simulink model "SNS_W2L_CPG"  (R2025b)
settings: Solver=ode1  StartTime=0.0  StopTime=10.0  FixedStep=0.002  RelTol=1e-3
libraries: SNS_Library x64
Description:
  | SNS_W2L_CPG: representative core of the W2L contact-driven bilateral CPG (build_w2l_net.py), SNS_Library blocks + custom NapHC (persistent Na, fixed tau_h). Validated against the numpy reference campaigns/20260930/w2l_numpy_ref.json.
settings Model: Creator=Ben  LastModifiedBy=Ben

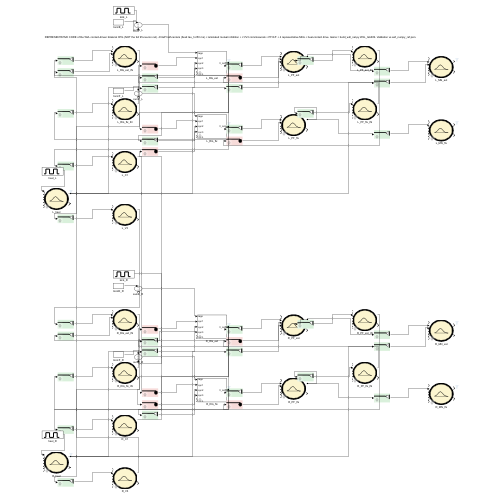
[thumbnail: Simulink's stored preview of the top-level diagram]
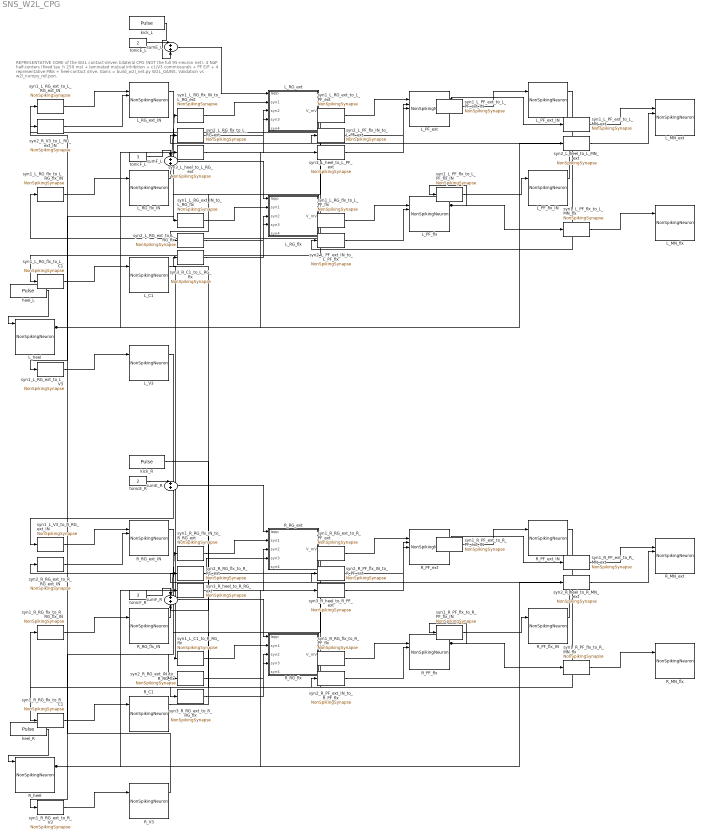
== system SNS_W2L_CPG ==
  note: REPRESENTATIVE CORE of the W2L contact-driven bilateral CPG (NOT the full 95-neuron net). 4 NaP half-centers (fixed tau_h 250 ms) + laminated mutual inhibition + c1/V3 commissurals + PF E/F + 4 representative MNs + heel-contact drive. Gains = build_w2l_net.py W2L_GAINS. Validation vs w2l_numpy_ref.json.
  L_C1 : SNS_Library/NonSpikingNeuron  Vrest=0  Gm=1  Cm=50  Thr=0  Slope=5
  L_MN_ext : SNS_Library/NonSpikingNeuron  Vrest=0  Gm=1  Cm=30  Thr=0  Slope=5
  L_MN_flx : SNS_Library/NonSpikingNeuron  Vrest=0  Gm=1  Cm=30  Thr=0  Slope=5
  L_PF_ext : SNS_Library/NonSpikingNeuron  Vrest=0  Gm=1  Cm=80  Thr=0  Slope=5
  L_PF_ext_IN : SNS_Library/NonSpikingNeuron  Vrest=0  Gm=1  Cm=80  Thr=0  Slope=5
  L_PF_flx : SNS_Library/NonSpikingNeuron  Vrest=0  Gm=1  Cm=80  Thr=0  Slope=5
  L_PF_flx_IN : SNS_Library/NonSpikingNeuron  Vrest=0  Gm=1  Cm=80  Thr=0  Slope=5
  L_RG_ext : Subsystem  mask{Vrest=0, Gm=1, Cm=50, GNa=12, ENa=8, kM=1, sM=0.8, eM=2, kH=1, sH=-2, eH=3.5, tauH=250, h0=0.9990889}
      mask prompts: Vrest "Resting potential Vrest (mV)"; Gm "Membrane conductance Gm (uS)"; Cm "Membrane capacitance Cm (nF)"; GNa "Persistent-Na conductance GNa (uS)"; ENa "Na reversal ENa (mV)"; kM "m-gate k"; sM "m-gate slope"; eM "m-gate midpoint (mV)"; kH "h-gate k"; sH "h-gate slope"; eH "h-gate midpoint (mV)"; tauH "h-gate time constant tauH (ms), FIXED"; h0 "initial h (h_inf(Vrest) for these params)"
      mask help: W2L persistent-Na half-center (sns_toolbox NonSpikingNeuronWithPersistentSodiumChannel semantics, FIXED tau_h). Cm dV/dt = Gm(Vrest-V) + Iapp + sum(g*Esyn) - V*sum(g) + GNa*m*h*(ENa-V); m = 1/(1+kM*exp(sM*(eM-V))); dh/dt = (hInf-h)/tauH with tauH FIXED (SNS_NumpyFixedTau / AnimatLab semantics). Params = spinal/params.py NAP with tau_max_h 0.25 s (build_w2l_net.py), membrane tau 50 ms.
  L_RG_ext_IN : SNS_Library/NonSpikingNeuron  Vrest=0  Gm=1  Cm=50  Thr=0  Slope=5
  L_RG_flx : Subsystem  mask{Vrest=0, Gm=1, Cm=50, GNa=12, ENa=8, kM=1, sM=0.8, eM=2, kH=1, sH=-2, eH=3.5, tauH=250, h0=0.9990889}
      mask prompts: Vrest "Resting potential Vrest (mV)"; Gm "Membrane conductance Gm (uS)"; Cm "Membrane capacitance Cm (nF)"; GNa "Persistent-Na conductance GNa (uS)"; ENa "Na reversal ENa (mV)"; kM "m-gate k"; sM "m-gate slope"; eM "m-gate midpoint (mV)"; kH "h-gate k"; sH "h-gate slope"; eH "h-gate midpoint (mV)"; tauH "h-gate time constant tauH (ms), FIXED"; h0 "initial h (h_inf(Vrest) for these params)"
      mask help: W2L persistent-Na half-center (sns_toolbox NonSpikingNeuronWithPersistentSodiumChannel semantics, FIXED tau_h). Cm dV/dt = Gm(Vrest-V) + Iapp + sum(g*Esyn) - V*sum(g) + GNa*m*h*(ENa-V); m = 1/(1+kM*exp(sM*(eM-V))); dh/dt = (hInf-h)/tauH with tauH FIXED (SNS_NumpyFixedTau / AnimatLab semantics). Params = spinal/params.py NAP with tau_max_h 0.25 s (build_w2l_net.py), membrane tau 50 ms.
  L_RG_flx_IN : SNS_Library/NonSpikingNeuron  Vrest=0  Gm=1  Cm=50  Thr=0  Slope=5
  L_V3 : SNS_Library/NonSpikingNeuron  Vrest=0  Gm=1  Cm=50  Thr=0  Slope=5
  L_heel : SNS_Library/NonSpikingNeuron  Vrest=0  Gm=1  Cm=40  Thr=0  Slope=5
  R_C1 : SNS_Library/NonSpikingNeuron  Vrest=0  Gm=1  Cm=50  Thr=0  Slope=5
  R_MN_ext : SNS_Library/NonSpikingNeuron  Vrest=0  Gm=1  Cm=30  Thr=0  Slope=5
  R_MN_flx : SNS_Library/NonSpikingNeuron  Vrest=0  Gm=1  Cm=30  Thr=0  Slope=5
  R_PF_ext : SNS_Library/NonSpikingNeuron  Vrest=0  Gm=1  Cm=80  Thr=0  Slope=5
  R_PF_ext_IN : SNS_Library/NonSpikingNeuron  Vrest=0  Gm=1  Cm=80  Thr=0  Slope=5
  R_PF_flx : SNS_Library/NonSpikingNeuron  Vrest=0  Gm=1  Cm=80  Thr=0  Slope=5
  R_PF_flx_IN : SNS_Library/NonSpikingNeuron  Vrest=0  Gm=1  Cm=80  Thr=0  Slope=5
  R_RG_ext : Subsystem  mask{Vrest=0, Gm=1, Cm=50, GNa=12, ENa=8, kM=1, sM=0.8, eM=2, kH=1, sH=-2, eH=3.5, tauH=250, h0=0.9990889}
      mask prompts: Vrest "Resting potential Vrest (mV)"; Gm "Membrane conductance Gm (uS)"; Cm "Membrane capacitance Cm (nF)"; GNa "Persistent-Na conductance GNa (uS)"; ENa "Na reversal ENa (mV)"; kM "m-gate k"; sM "m-gate slope"; eM "m-gate midpoint (mV)"; kH "h-gate k"; sH "h-gate slope"; eH "h-gate midpoint (mV)"; tauH "h-gate time constant tauH (ms), FIXED"; h0 "initial h (h_inf(Vrest) for these params)"
      mask help: W2L persistent-Na half-center (sns_toolbox NonSpikingNeuronWithPersistentSodiumChannel semantics, FIXED tau_h). Cm dV/dt = Gm(Vrest-V) + Iapp + sum(g*Esyn) - V*sum(g) + GNa*m*h*(ENa-V); m = 1/(1+kM*exp(sM*(eM-V))); dh/dt = (hInf-h)/tauH with tauH FIXED (SNS_NumpyFixedTau / AnimatLab semantics). Params = spinal/params.py NAP with tau_max_h 0.25 s (build_w2l_net.py), membrane tau 50 ms.
  R_RG_ext_IN : SNS_Library/NonSpikingNeuron  Vrest=0  Gm=1  Cm=50  Thr=0  Slope=5
  R_RG_flx : Subsystem  mask{Vrest=0, Gm=1, Cm=50, GNa=12, ENa=8, kM=1, sM=0.8, eM=2, kH=1, sH=-2, eH=3.5, tauH=250, h0=0.9990889}
      mask prompts: Vrest "Resting potential Vrest (mV)"; Gm "Membrane conductance Gm (uS)"; Cm "Membrane capacitance Cm (nF)"; GNa "Persistent-Na conductance GNa (uS)"; ENa "Na reversal ENa (mV)"; kM "m-gate k"; sM "m-gate slope"; eM "m-gate midpoint (mV)"; kH "h-gate k"; sH "h-gate slope"; eH "h-gate midpoint (mV)"; tauH "h-gate time constant tauH (ms), FIXED"; h0 "initial h (h_inf(Vrest) for these params)"
      mask help: W2L persistent-Na half-center (sns_toolbox NonSpikingNeuronWithPersistentSodiumChannel semantics, FIXED tau_h). Cm dV/dt = Gm(Vrest-V) + Iapp + sum(g*Esyn) - V*sum(g) + GNa*m*h*(ENa-V); m = 1/(1+kM*exp(sM*(eM-V))); dh/dt = (hInf-h)/tauH with tauH FIXED (SNS_NumpyFixedTau / AnimatLab semantics). Params = spinal/params.py NAP with tau_max_h 0.25 s (build_w2l_net.py), membrane tau 50 ms.
  R_RG_flx_IN : SNS_Library/NonSpikingNeuron  Vrest=0  Gm=1  Cm=50  Thr=0  Slope=5
  R_V3 : SNS_Library/NonSpikingNeuron  Vrest=0  Gm=1  Cm=50  Thr=0  Slope=5
  R_heel : SNS_Library/NonSpikingNeuron  Vrest=0  Gm=1  Cm=40  Thr=0  Slope=5
  heel_L : DiscretePulseGenerator  PulseType=Time based  Amplitude=20  Period=1  PulseWidth=30
  heel_R : DiscretePulseGenerator  PulseType=Time based  Amplitude=20  Period=1  PulseWidth=30  PhaseDelay=0.5
  kick_L : DiscretePulseGenerator  PulseType=Time based  Amplitude=10  Period=24  PulseWidth=0.04166666667
  kick_R : DiscretePulseGenerator  PulseType=Time based  Amplitude=10  Period=24  PulseWidth=0.04166666667
  sumE_L : Sum
  sumE_R : Sum
  sumF_L : Sum
  sumF_R : Sum
  syn1_L_C1_to_R_RG_flx : SNS_Library/NonSpikingSynapse  gmax=3  Esyn=-5  ThrPre=0  SlopePre=5
  syn1_L_PF_ext_to_L_MN_ext : SNS_Library/NonSpikingSynapse  gmax=2  Esyn=8  ThrPre=0  SlopePre=5
  syn1_L_PF_ext_to_L_PF_ext_IN : SNS_Library/NonSpikingSynapse  gmax=4  Esyn=8  ThrPre=0  SlopePre=5
  syn1_L_PF_flx_to_L_MN_flx : SNS_Library/NonSpikingSynapse  gmax=2  Esyn=8  ThrPre=0  SlopePre=5
  syn1_L_PF_flx_to_L_PF_flx_IN : SNS_Library/NonSpikingSynapse  gmax=4  Esyn=8  ThrPre=0  SlopePre=5
  syn1_L_RG_ext_IN_to_L_RG_flx : SNS_Library/NonSpikingSynapse  gmax=4  Esyn=-5  ThrPre=0  SlopePre=5
  syn1_L_RG_ext_to_L_PF_ext : SNS_Library/NonSpikingSynapse  gmax=2.4  Esyn=8  ThrPre=0  SlopePre=5
  syn1_L_RG_ext_to_L_RG_ext_IN : SNS_Library/NonSpikingSynapse  gmax=4  Esyn=8  ThrPre=0  SlopePre=5
  syn1_L_RG_ext_to_L_V3 : SNS_Library/NonSpikingSynapse  gmax=1  Esyn=8  ThrPre=0  SlopePre=5
  syn1_L_RG_flx_IN_to_L_RG_ext : SNS_Library/NonSpikingSynapse  gmax=4  Esyn=-5  ThrPre=0  SlopePre=5
  syn1_L_RG_flx_to_L_C1 : SNS_Library/NonSpikingSynapse  gmax=1  Esyn=8  ThrPre=0  SlopePre=5
  syn1_L_RG_flx_to_L_PF_flx : SNS_Library/NonSpikingSynapse  gmax=2.4  Esyn=8  ThrPre=0  SlopePre=5
  syn1_L_RG_flx_to_L_RG_flx_IN : SNS_Library/NonSpikingSynapse  gmax=4  Esyn=8  ThrPre=0  SlopePre=5
  syn1_L_V3_to_R_RG_ext_IN : SNS_Library/NonSpikingSynapse  gmax=0.08  Esyn=8  ThrPre=0  SlopePre=5
  syn1_R_PF_ext_to_R_MN_ext : SNS_Library/NonSpikingSynapse  gmax=2  Esyn=8  ThrPre=0  SlopePre=5
  syn1_R_PF_ext_to_R_PF_ext_IN : SNS_Library/NonSpikingSynapse  gmax=4  Esyn=8  ThrPre=0  SlopePre=5
  syn1_R_PF_flx_to_R_MN_flx : SNS_Library/NonSpikingSynapse  gmax=2  Esyn=8  ThrPre=0  SlopePre=5
  syn1_R_PF_flx_to_R_PF_flx_IN : SNS_Library/NonSpikingSynapse  gmax=4  Esyn=8  ThrPre=0  SlopePre=5
  syn1_R_RG_ext_to_R_PF_ext : SNS_Library/NonSpikingSynapse  gmax=2.4  Esyn=8  ThrPre=0  SlopePre=5
  syn1_R_RG_ext_to_R_V3 : SNS_Library/NonSpikingSynapse  gmax=1  Esyn=8  ThrPre=0  SlopePre=5
  syn1_R_RG_flx_IN_to_R_RG_ext : SNS_Library/NonSpikingSynapse  gmax=4  Esyn=-5  ThrPre=0  SlopePre=5
  syn1_R_RG_flx_to_R_C1 : SNS_Library/NonSpikingSynapse  gmax=1  Esyn=8  ThrPre=0  SlopePre=5
  syn1_R_RG_flx_to_R_PF_flx : SNS_Library/NonSpikingSynapse  gmax=2.4  Esyn=8  ThrPre=0  SlopePre=5
  syn1_R_RG_flx_to_R_RG_flx_IN : SNS_Library/NonSpikingSynapse  gmax=4  Esyn=8  ThrPre=0  SlopePre=5
  syn2_L_PF_ext_IN_to_L_PF_flx : SNS_Library/NonSpikingSynapse  gmax=4  Esyn=-5  ThrPre=0  SlopePre=5
  syn2_L_PF_flx_IN_to_L_PF_ext : SNS_Library/NonSpikingSynapse  gmax=4  Esyn=-5  ThrPre=0  SlopePre=5
  syn2_L_RG_ext_to_L_RG_flx : SNS_Library/NonSpikingSynapse  gmax=0.5  Esyn=8  ThrPre=0  SlopePre=5
  syn2_L_RG_flx_to_L_RG_ext : SNS_Library/NonSpikingSynapse  gmax=0.5  Esyn=8  ThrPre=0  SlopePre=5
  syn2_L_heel_to_L_MN_ext : SNS_Library/NonSpikingSynapse  gmax=1  Esyn=8  ThrPre=0  SlopePre=5
  syn2_R_PF_ext_IN_to_R_PF_flx : SNS_Library/NonSpikingSynapse  gmax=4  Esyn=-5  ThrPre=0  SlopePre=5
  syn2_R_PF_flx_IN_to_R_PF_ext : SNS_Library/NonSpikingSynapse  gmax=4  Esyn=-5  ThrPre=0  SlopePre=5
  syn2_R_RG_ext_IN_to_R_RG_flx : SNS_Library/NonSpikingSynapse  gmax=4  Esyn=-5  ThrPre=0  SlopePre=5
  syn2_R_RG_ext_to_R_RG_ext_IN : SNS_Library/NonSpikingSynapse  gmax=4  Esyn=8  ThrPre=0  SlopePre=5
  syn2_R_RG_flx_to_R_RG_ext : SNS_Library/NonSpikingSynapse  gmax=0.5  Esyn=8  ThrPre=0  SlopePre=5
  syn2_R_V3_to_L_RG_ext_IN : SNS_Library/NonSpikingSynapse  gmax=0.08  Esyn=8  ThrPre=0  SlopePre=5
  syn2_R_heel_to_R_MN_ext : SNS_Library/NonSpikingSynapse  gmax=1  Esyn=8  ThrPre=0  SlopePre=5
  syn3_L_heel_to_L_PF_ext : SNS_Library/NonSpikingSynapse  gmax=1  Esyn=8  ThrPre=0  SlopePre=5
  syn3_L_heel_to_L_RG_ext : SNS_Library/NonSpikingSynapse  gmax=1  Esyn=8  ThrPre=0  SlopePre=5
  syn3_R_C1_to_L_RG_flx : SNS_Library/NonSpikingSynapse  gmax=3  Esyn=-5  ThrPre=0  SlopePre=5
  syn3_R_RG_ext_to_R_RG_flx : SNS_Library/NonSpikingSynapse  gmax=0.5  Esyn=8  ThrPre=0  SlopePre=5
  syn3_R_heel_to_R_PF_ext : SNS_Library/NonSpikingSynapse  gmax=1  Esyn=8  ThrPre=0  SlopePre=5
  syn3_R_heel_to_R_RG_ext : SNS_Library/NonSpikingSynapse  gmax=1  Esyn=8  ThrPre=0  SlopePre=5
  tonicE_L : Constant  Value=2
  tonicE_R : Constant  Value=2
  tonicF_L : Constant  Value=3
  tonicF_R : Constant  Value=3
  wires:
  L_RG_ext/1(V_mV) -> syn1_L_RG_ext_to_L_RG_ext_IN/1, syn2_L_RG_ext_to_L_RG_flx/1, syn1_L_RG_ext_to_L_V3/1, syn1_L_RG_ext_to_L_PF_ext/1
  syn1_L_RG_ext_to_L_RG_ext_IN/1 -> L_RG_ext_IN/2
  L_RG_ext_IN/1 -> syn1_L_RG_ext_IN_to_L_RG_flx/1
  syn1_L_RG_ext_IN_to_L_RG_flx/1 -> L_RG_flx/2(syn1)
  L_RG_flx/1(V_mV) -> syn1_L_RG_flx_to_L_RG_flx_IN/1, syn2_L_RG_flx_to_L_RG_ext/1, syn1_L_RG_flx_to_L_C1/1, syn1_L_RG_flx_to_L_PF_flx/1
  syn1_L_RG_flx_to_L_RG_flx_IN/1 -> L_RG_flx_IN/2
  L_RG_flx_IN/1 -> syn1_L_RG_flx_IN_to_L_RG_ext/1
  syn1_L_RG_flx_IN_to_L_RG_ext/1 -> L_RG_ext/2(syn1)
  syn2_L_RG_ext_to_L_RG_flx/1 -> L_RG_flx/3(syn2)
  syn2_L_RG_flx_to_L_RG_ext/1 -> L_RG_ext/3(syn2)
  syn1_L_RG_flx_to_L_C1/1 -> L_C1/2
  L_C1/1 -> syn1_L_C1_to_R_RG_flx/1
  syn1_L_C1_to_R_RG_flx/1 -> R_RG_flx/2(syn1)
  syn1_L_RG_ext_to_L_V3/1 -> L_V3/2
  L_V3/1 -> syn1_L_V3_to_R_RG_ext_IN/1
  syn1_L_V3_to_R_RG_ext_IN/1 -> R_RG_ext_IN/2
  syn1_L_RG_ext_to_L_PF_ext/1 -> L_PF_ext/2
  syn1_L_RG_flx_to_L_PF_flx/1 -> L_PF_flx/2
  L_PF_ext/1 -> syn1_L_PF_ext_to_L_PF_ext_IN/1, syn1_L_PF_ext_to_L_MN_ext/1
  syn1_L_PF_ext_to_L_PF_ext_IN/1 -> L_PF_ext_IN/2
  L_PF_ext_IN/1 -> syn2_L_PF_ext_IN_to_L_PF_flx/1
  syn2_L_PF_ext_IN_to_L_PF_flx/1 -> L_PF_flx/3
  L_PF_flx/1 -> syn1_L_PF_flx_to_L_PF_flx_IN/1, syn1_L_PF_flx_to_L_MN_flx/1
  syn1_L_PF_flx_to_L_PF_flx_IN/1 -> L_PF_flx_IN/2
  L_PF_flx_IN/1 -> syn2_L_PF_flx_IN_to_L_PF_ext/1
  syn2_L_PF_flx_IN_to_L_PF_ext/1 -> L_PF_ext/3
  syn1_L_PF_ext_to_L_MN_ext/1 -> L_MN_ext/2
  syn1_L_PF_flx_to_L_MN_flx/1 -> L_MN_flx/2
  L_heel/1 -> syn3_L_heel_to_L_RG_ext/1, syn3_L_heel_to_L_PF_ext/1, syn2_L_heel_to_L_MN_ext/1
  syn3_L_heel_to_L_RG_ext/1 -> L_RG_ext/4(syn3)
  syn3_L_heel_to_L_PF_ext/1 -> L_PF_ext/4
  syn2_L_heel_to_L_MN_ext/1 -> L_MN_ext/3
  R_RG_ext/1(V_mV) -> syn2_R_RG_ext_to_R_RG_ext_IN/1, syn3_R_RG_ext_to_R_RG_flx/1, syn1_R_RG_ext_to_R_V3/1, syn1_R_RG_ext_to_R_PF_ext/1
  syn2_R_RG_ext_to_R_RG_ext_IN/1 -> R_RG_ext_IN/3
  R_RG_ext_IN/1 -> syn2_R_RG_ext_IN_to_R_RG_flx/1
  syn2_R_RG_ext_IN_to_R_RG_flx/1 -> R_RG_flx/3(syn2)
  R_RG_flx/1(V_mV) -> syn1_R_RG_flx_to_R_RG_flx_IN/1, syn2_R_RG_flx_to_R_RG_ext/1, syn1_R_RG_flx_to_R_C1/1, syn1_R_RG_flx_to_R_PF_flx/1
  syn1_R_RG_flx_to_R_RG_flx_IN/1 -> R_RG_flx_IN/2
  R_RG_flx_IN/1 -> syn1_R_RG_flx_IN_to_R_RG_ext/1
  syn1_R_RG_flx_IN_to_R_RG_ext/1 -> R_RG_ext/2(syn1)
  syn3_R_RG_ext_to_R_RG_flx/1 -> R_RG_flx/4(syn3)
  syn2_R_RG_flx_to_R_RG_ext/1 -> R_RG_ext/3(syn2)
  syn1_R_RG_flx_to_R_C1/1 -> R_C1/2
  R_C1/1 -> syn3_R_C1_to_L_RG_flx/1
  syn3_R_C1_to_L_RG_flx/1 -> L_RG_flx/4(syn3)
  syn1_R_RG_ext_to_R_V3/1 -> R_V3/2
  R_V3/1 -> syn2_R_V3_to_L_RG_ext_IN/1
  syn2_R_V3_to_L_RG_ext_IN/1 -> L_RG_ext_IN/3
  syn1_R_RG_ext_to_R_PF_ext/1 -> R_PF_ext/2
  syn1_R_RG_flx_to_R_PF_flx/1 -> R_PF_flx/2
  R_PF_ext/1 -> syn1_R_PF_ext_to_R_PF_ext_IN/1, syn1_R_PF_ext_to_R_MN_ext/1
  syn1_R_PF_ext_to_R_PF_ext_IN/1 -> R_PF_ext_IN/2
  R_PF_ext_IN/1 -> syn2_R_PF_ext_IN_to_R_PF_flx/1
  syn2_R_PF_ext_IN_to_R_PF_flx/1 -> R_PF_flx/3
  R_PF_flx/1 -> syn1_R_PF_flx_to_R_PF_flx_IN/1, syn1_R_PF_flx_to_R_MN_flx/1
  syn1_R_PF_flx_to_R_PF_flx_IN/1 -> R_PF_flx_IN/2
  R_PF_flx_IN/1 -> syn2_R_PF_flx_IN_to_R_PF_ext/1
  syn2_R_PF_flx_IN_to_R_PF_ext/1 -> R_PF_ext/3
  syn1_R_PF_ext_to_R_MN_ext/1 -> R_MN_ext/2
  syn1_R_PF_flx_to_R_MN_flx/1 -> R_MN_flx/2
  R_heel/1 -> syn3_R_heel_to_R_RG_ext/1, syn3_R_heel_to_R_PF_ext/1, syn2_R_heel_to_R_MN_ext/1
  syn3_R_heel_to_R_RG_ext/1 -> R_RG_ext/4(syn3)
  syn3_R_heel_to_R_PF_ext/1 -> R_PF_ext/4
  syn2_R_heel_to_R_MN_ext/1 -> R_MN_ext/3
  tonicE_L/1 -> sumE_L/1
  tonicF_L/1 -> sumF_L/1
  sumE_L/1 -> L_RG_ext/1(Iapp)
  sumF_L/1 -> L_RG_flx/1(Iapp)
  heel_L/1 -> L_heel/1
  tonicE_R/1 -> sumE_R/1
  tonicF_R/1 -> sumF_R/1
  sumE_R/1 -> R_RG_ext/1(Iapp)
  sumF_R/1 -> R_RG_flx/1(Iapp)
  heel_R/1 -> R_heel/1
  kick_L/1 -> sumE_L/2
  kick_R/1 -> sumF_R/2

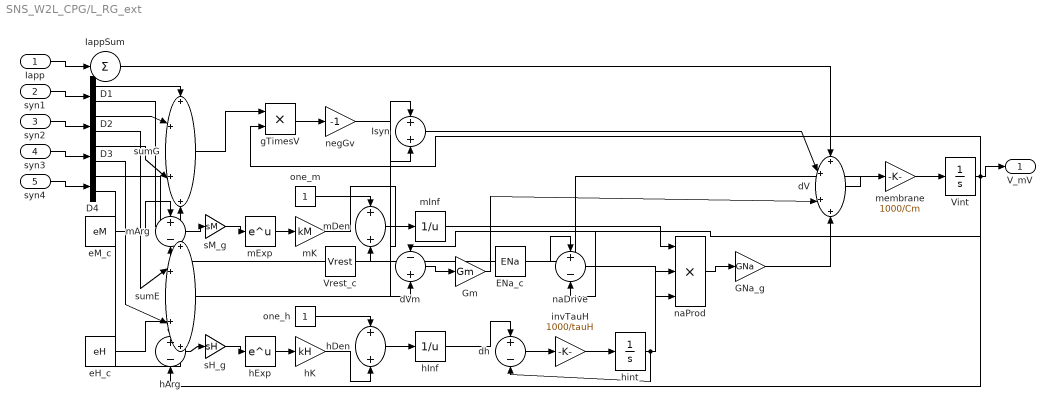
== system SNS_W2L_CPG/L_RG_ext ==
  Iapp : Inport
  syn1 : Inport  Port=2  PortDimensions=2
  syn2 : Inport  Port=3  PortDimensions=2
  syn3 : Inport  Port=4  PortDimensions=2
  syn4 : Inport  Port=5  PortDimensions=2
  D{1..4} (4 alike) : Demux  Outputs=2
  ENa_c : Constant  Value=ENa
  GNa_g : Gain  Gain=GNa
  Gm : Gain  Gain=Gm
  IappSum : Sum  Inputs=+
  Isyn : Sum
  Vint : Integrator  InitialCondition=Vrest
  Vrest_c : Constant  Value=Vrest
  dV : Sum  Inputs=++++
  dVm : Sum  Inputs=-+
  dh : Sum  Inputs=+-
  eH_c : Constant  Value=eH
  eM_c : Constant  Value=eM
  gTimesV : Product
  hArg : Sum  Inputs=+-
  hDen : Sum
  hExp : Math
  hInf : Math  Operator=reciprocal
  hK : Gain  Gain=kH
  hint : Integrator  InitialCondition=h0
  invTauH : Gain  Gain=1000/tauH
  mArg : Sum  Inputs=+-
  mDen : Sum
  mExp : Math
  mInf : Math  Operator=reciprocal
  mK : Gain  Gain=kM
  membrane : Gain  Gain=1000/Cm
  naDrive : Sum  Inputs=+-
  naProd : Product  Inputs=3
  negGv : Gain  Gain=-1
  one_h : Constant
  one_m : Constant
  sH_g : Gain  Gain=sH
  sM_g : Gain  Gain=sM
  sumE : Sum  Inputs=++++
  sumG : Sum  Inputs=++++
  V_mV : Outport
  wires:
  Vint/1 -> naDrive/2, hArg/2, mArg/2, dVm/1, gTimesV/2, V_mV/1
  membrane/1 -> Vint/1
  dV/1 -> membrane/1
  GNa_g/1 -> dV/4
  Gm/1 -> dV/3
  Isyn/1 -> dV/2
  IappSum/1 -> dV/1
  Iapp/1 -> IappSum/1
  naProd/1 -> GNa_g/1
  naDrive/1 -> naProd/3
  mInf/1 -> naProd/1
  ENa_c/1 -> naDrive/1
  invTauH/1 -> hint/1
  dh/1 -> invTauH/1
  hint/1 -> naProd/2, dh/2
  hInf/1 -> dh/1
  hDen/1 -> hInf/1
  hK/1 -> hDen/2
  one_h/1 -> hDen/1
  hExp/1 -> hK/1
  sH_g/1 -> hExp/1
  hArg/1 -> sH_g/1
  eH_c/1 -> hArg/1
  mDen/1 -> mInf/1
  mK/1 -> mDen/2
  one_m/1 -> mDen/1
  mExp/1 -> mK/1
  sM_g/1 -> mExp/1
  mArg/1 -> sM_g/1
  eM_c/1 -> mArg/1
  dVm/1 -> Gm/1
  Vrest_c/1 -> dVm/2
  negGv/1 -> Isyn/2
  sumE/1 -> Isyn/1
  gTimesV/1 -> negGv/1
  sumG/1 -> gTimesV/1
  D4/2 -> sumE/4
  D4/1 -> sumG/4
  D3/2 -> sumE/3
  D3/1 -> sumG/3
  D2/2 -> sumE/2
  D2/1 -> sumG/2
  D1/2 -> sumE/1
  D1/1 -> sumG/1
  syn4/1 -> D4/1
  syn3/1 -> D3/1
  syn2/1 -> D2/1
  syn1/1 -> D1/1

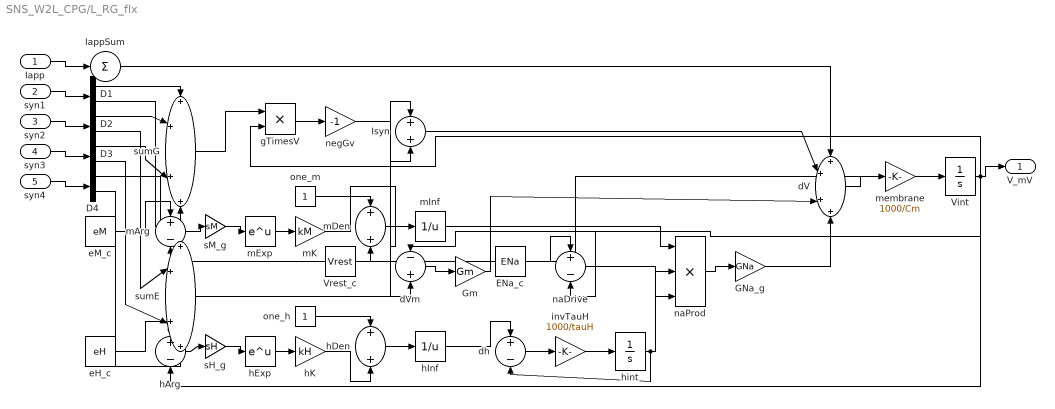
== system SNS_W2L_CPG/L_RG_flx ==
  Iapp : Inport
  syn1 : Inport  Port=2  PortDimensions=2
  syn2 : Inport  Port=3  PortDimensions=2
  syn3 : Inport  Port=4  PortDimensions=2
  syn4 : Inport  Port=5  PortDimensions=2
  D{1..4} (4 alike) : Demux  Outputs=2
  ENa_c : Constant  Value=ENa
  GNa_g : Gain  Gain=GNa
  Gm : Gain  Gain=Gm
  IappSum : Sum  Inputs=+
  Isyn : Sum
  Vint : Integrator  InitialCondition=Vrest
  Vrest_c : Constant  Value=Vrest
  dV : Sum  Inputs=++++
  dVm : Sum  Inputs=-+
  dh : Sum  Inputs=+-
  eH_c : Constant  Value=eH
  eM_c : Constant  Value=eM
  gTimesV : Product
  hArg : Sum  Inputs=+-
  hDen : Sum
  hExp : Math
  hInf : Math  Operator=reciprocal
  hK : Gain  Gain=kH
  hint : Integrator  InitialCondition=h0
  invTauH : Gain  Gain=1000/tauH
  mArg : Sum  Inputs=+-
  mDen : Sum
  mExp : Math
  mInf : Math  Operator=reciprocal
  mK : Gain  Gain=kM
  membrane : Gain  Gain=1000/Cm
  naDrive : Sum  Inputs=+-
  naProd : Product  Inputs=3
  negGv : Gain  Gain=-1
  one_h : Constant
  one_m : Constant
  sH_g : Gain  Gain=sH
  sM_g : Gain  Gain=sM
  sumE : Sum  Inputs=++++
  sumG : Sum  Inputs=++++
  V_mV : Outport
  wires:
  Vint/1 -> naDrive/2, hArg/2, mArg/2, dVm/1, gTimesV/2, V_mV/1
  membrane/1 -> Vint/1
  dV/1 -> membrane/1
  GNa_g/1 -> dV/4
  Gm/1 -> dV/3
  Isyn/1 -> dV/2
  IappSum/1 -> dV/1
  Iapp/1 -> IappSum/1
  naProd/1 -> GNa_g/1
  naDrive/1 -> naProd/3
  mInf/1 -> naProd/1
  ENa_c/1 -> naDrive/1
  invTauH/1 -> hint/1
  dh/1 -> invTauH/1
  hint/1 -> naProd/2, dh/2
  hInf/1 -> dh/1
  hDen/1 -> hInf/1
  hK/1 -> hDen/2
  one_h/1 -> hDen/1
  hExp/1 -> hK/1
  sH_g/1 -> hExp/1
  hArg/1 -> sH_g/1
  eH_c/1 -> hArg/1
  mDen/1 -> mInf/1
  mK/1 -> mDen/2
  one_m/1 -> mDen/1
  mExp/1 -> mK/1
  sM_g/1 -> mExp/1
  mArg/1 -> sM_g/1
  eM_c/1 -> mArg/1
  dVm/1 -> Gm/1
  Vrest_c/1 -> dVm/2
  negGv/1 -> Isyn/2
  sumE/1 -> Isyn/1
  gTimesV/1 -> negGv/1
  sumG/1 -> gTimesV/1
  D4/2 -> sumE/4
  D4/1 -> sumG/4
  D3/2 -> sumE/3
  D3/1 -> sumG/3
  D2/2 -> sumE/2
  D2/1 -> sumG/2
  D1/2 -> sumE/1
  D1/1 -> sumG/1
  syn4/1 -> D4/1
  syn3/1 -> D3/1
  syn2/1 -> D2/1
  syn1/1 -> D1/1

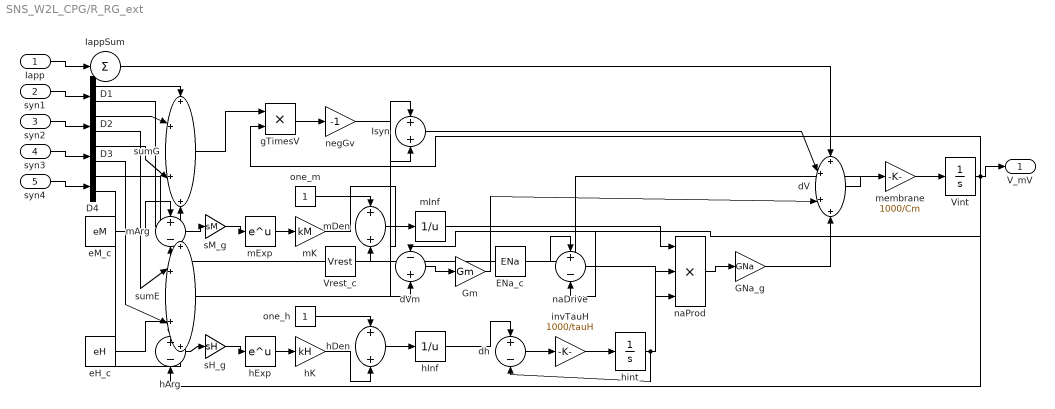
== system SNS_W2L_CPG/R_RG_ext ==
  Iapp : Inport
  syn1 : Inport  Port=2  PortDimensions=2
  syn2 : Inport  Port=3  PortDimensions=2
  syn3 : Inport  Port=4  PortDimensions=2
  syn4 : Inport  Port=5  PortDimensions=2
  D{1..4} (4 alike) : Demux  Outputs=2
  ENa_c : Constant  Value=ENa
  GNa_g : Gain  Gain=GNa
  Gm : Gain  Gain=Gm
  IappSum : Sum  Inputs=+
  Isyn : Sum
  Vint : Integrator  InitialCondition=Vrest
  Vrest_c : Constant  Value=Vrest
  dV : Sum  Inputs=++++
  dVm : Sum  Inputs=-+
  dh : Sum  Inputs=+-
  eH_c : Constant  Value=eH
  eM_c : Constant  Value=eM
  gTimesV : Product
  hArg : Sum  Inputs=+-
  hDen : Sum
  hExp : Math
  hInf : Math  Operator=reciprocal
  hK : Gain  Gain=kH
  hint : Integrator  InitialCondition=h0
  invTauH : Gain  Gain=1000/tauH
  mArg : Sum  Inputs=+-
  mDen : Sum
  mExp : Math
  mInf : Math  Operator=reciprocal
  mK : Gain  Gain=kM
  membrane : Gain  Gain=1000/Cm
  naDrive : Sum  Inputs=+-
  naProd : Product  Inputs=3
  negGv : Gain  Gain=-1
  one_h : Constant
  one_m : Constant
  sH_g : Gain  Gain=sH
  sM_g : Gain  Gain=sM
  sumE : Sum  Inputs=++++
  sumG : Sum  Inputs=++++
  V_mV : Outport
  wires:
  Vint/1 -> naDrive/2, hArg/2, mArg/2, dVm/1, gTimesV/2, V_mV/1
  membrane/1 -> Vint/1
  dV/1 -> membrane/1
  GNa_g/1 -> dV/4
  Gm/1 -> dV/3
  Isyn/1 -> dV/2
  IappSum/1 -> dV/1
  Iapp/1 -> IappSum/1
  naProd/1 -> GNa_g/1
  naDrive/1 -> naProd/3
  mInf/1 -> naProd/1
  ENa_c/1 -> naDrive/1
  invTauH/1 -> hint/1
  dh/1 -> invTauH/1
  hint/1 -> naProd/2, dh/2
  hInf/1 -> dh/1
  hDen/1 -> hInf/1
  hK/1 -> hDen/2
  one_h/1 -> hDen/1
  hExp/1 -> hK/1
  sH_g/1 -> hExp/1
  hArg/1 -> sH_g/1
  eH_c/1 -> hArg/1
  mDen/1 -> mInf/1
  mK/1 -> mDen/2
  one_m/1 -> mDen/1
  mExp/1 -> mK/1
  sM_g/1 -> mExp/1
  mArg/1 -> sM_g/1
  eM_c/1 -> mArg/1
  dVm/1 -> Gm/1
  Vrest_c/1 -> dVm/2
  negGv/1 -> Isyn/2
  sumE/1 -> Isyn/1
  gTimesV/1 -> negGv/1
  sumG/1 -> gTimesV/1
  D4/2 -> sumE/4
  D4/1 -> sumG/4
  D3/2 -> sumE/3
  D3/1 -> sumG/3
  D2/2 -> sumE/2
  D2/1 -> sumG/2
  D1/2 -> sumE/1
  D1/1 -> sumG/1
  syn4/1 -> D4/1
  syn3/1 -> D3/1
  syn2/1 -> D2/1
  syn1/1 -> D1/1

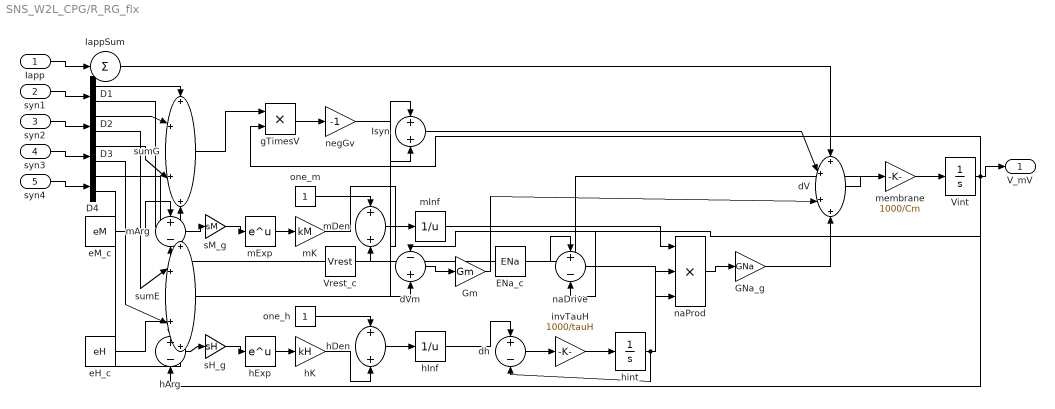
== system SNS_W2L_CPG/R_RG_flx ==
  Iapp : Inport
  syn1 : Inport  Port=2  PortDimensions=2
  syn2 : Inport  Port=3  PortDimensions=2
  syn3 : Inport  Port=4  PortDimensions=2
  syn4 : Inport  Port=5  PortDimensions=2
  D{1..4} (4 alike) : Demux  Outputs=2
  ENa_c : Constant  Value=ENa
  GNa_g : Gain  Gain=GNa
  Gm : Gain  Gain=Gm
  IappSum : Sum  Inputs=+
  Isyn : Sum
  Vint : Integrator  InitialCondition=Vrest
  Vrest_c : Constant  Value=Vrest
  dV : Sum  Inputs=++++
  dVm : Sum  Inputs=-+
  dh : Sum  Inputs=+-
  eH_c : Constant  Value=eH
  eM_c : Constant  Value=eM
  gTimesV : Product
  hArg : Sum  Inputs=+-
  hDen : Sum
  hExp : Math
  hInf : Math  Operator=reciprocal
  hK : Gain  Gain=kH
  hint : Integrator  InitialCondition=h0
  invTauH : Gain  Gain=1000/tauH
  mArg : Sum  Inputs=+-
  mDen : Sum
  mExp : Math
  mInf : Math  Operator=reciprocal
  mK : Gain  Gain=kM
  membrane : Gain  Gain=1000/Cm
  naDrive : Sum  Inputs=+-
  naProd : Product  Inputs=3
  negGv : Gain  Gain=-1
  one_h : Constant
  one_m : Constant
  sH_g : Gain  Gain=sH
  sM_g : Gain  Gain=sM
  sumE : Sum  Inputs=++++
  sumG : Sum  Inputs=++++
  V_mV : Outport
  wires:
  Vint/1 -> naDrive/2, hArg/2, mArg/2, dVm/1, gTimesV/2, V_mV/1
  membrane/1 -> Vint/1
  dV/1 -> membrane/1
  GNa_g/1 -> dV/4
  Gm/1 -> dV/3
  Isyn/1 -> dV/2
  IappSum/1 -> dV/1
  Iapp/1 -> IappSum/1
  naProd/1 -> GNa_g/1
  naDrive/1 -> naProd/3
  mInf/1 -> naProd/1
  ENa_c/1 -> naDrive/1
  invTauH/1 -> hint/1
  dh/1 -> invTauH/1
  hint/1 -> naProd/2, dh/2
  hInf/1 -> dh/1
  hDen/1 -> hInf/1
  hK/1 -> hDen/2
  one_h/1 -> hDen/1
  hExp/1 -> hK/1
  sH_g/1 -> hExp/1
  hArg/1 -> sH_g/1
  eH_c/1 -> hArg/1
  mDen/1 -> mInf/1
  mK/1 -> mDen/2
  one_m/1 -> mDen/1
  mExp/1 -> mK/1
  sM_g/1 -> mExp/1
  mArg/1 -> sM_g/1
  eM_c/1 -> mArg/1
  dVm/1 -> Gm/1
  Vrest_c/1 -> dVm/2
  negGv/1 -> Isyn/2
  sumE/1 -> Isyn/1
  gTimesV/1 -> negGv/1
  sumG/1 -> gTimesV/1
  D4/2 -> sumE/4
  D4/1 -> sumG/4
  D3/2 -> sumE/3
  D3/1 -> sumG/3
  D2/2 -> sumE/2
  D2/1 -> sumG/2
  D1/2 -> sumE/1
  D1/1 -> sumG/1
  syn4/1 -> D4/1
  syn3/1 -> D3/1
  syn2/1 -> D2/1
  syn1/1 -> D1/1
